simulink model "MATLABxuexiduanluqi"  (R2016a)
settings: Solver=VariableStepAuto  StartTime=0.0  StopTime=0.7  RelTol=1e-3
libraries: powerlib x12
settings Model: Creator=24535  LastModifiedBy=24535

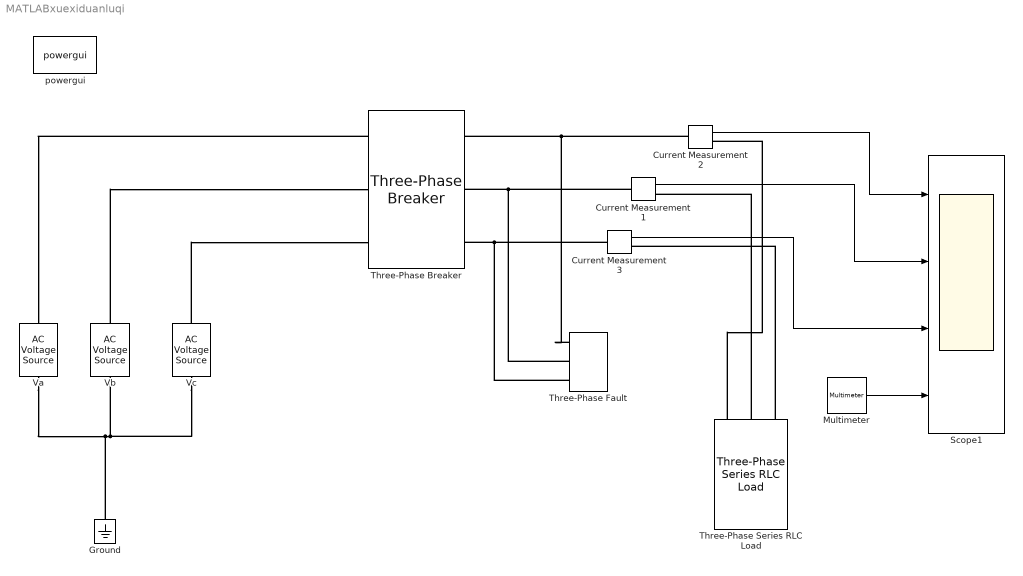
== system MATLABxuexiduanluqi ==
  Current Measurement1 : powerlib/Measurements/Current Measurement  PhasorSimulation=off  OutputType=Complex  PSBequivalent=0
  Current Measurement2 : powerlib/Measurements/Current Measurement  PhasorSimulation=off  OutputType=Complex  PSBequivalent=0
  Current Measurement3 : powerlib/Measurements/Current Measurement  PhasorSimulation=off  OutputType=Complex  PSBequivalent=0
  Ground : powerlib/Elements/Ground  LConnTagsString=a
  Multimeter : powerlib/Measurements/Multimeter  PhasorSimulation=off  OutputType=Complex  sel=7  L=9  Gain=1  yselected={'Ib: Three-Phase Fault/Fault A'};  PSBOutputType=1  PSBequivalent=0  AxesSetting=[0,0.1,-100,100]  Display=0  SavedBlockNames=-11
  Scope1 : Scope  NumInputPorts=4
  Three-Phase Series RLC Load : powerlib/Elements/Three-Phase Series RLC Load  LConnTagsString=A|B|C  Configuration=Y (grounded)  NominalVoltage=5000  Vabc=[1e3 1e3 1e3]  Vabcp=[1e3 1e3 1e3]  NominalFrequency=50  UnbalancedPower=off  ActivePower=1000  InductivePower=330  CapacitivePower=0  Pabc=[10e3 9e3 11e3]  QLabc=[100 90 110]  QCabc=[100 90 110]  Pabcp=[10e3 9e3 11e3]  QLabcp=[100 90 110]  QCabcp=[100 90 110]  Measurements=Branch voltages  LoadType=constant Z
  Three-Phase Breaker : powerlib/Elements/Three-Phase Breaker  InitialState=open  SwitchA=on  SwitchB=on  SwitchC=on  SwitchTimes="[1/50  0.4]"  External=off  BreakerResistance=0.01  SnubberResistance=100  SnubberCapacitance=0.47e-6  Measurements=None
  Three-Phase Fault : powerlib/Elements/Three-Phase Fault  InitialStates=0  FaultA=on  FaultB=on  FaultC=on  GroundFault=on  SwitchTimes="[1/10  3/5]"  External=off  SwitchStatus=NaN  FaultResistance=0.001  GroundResistance=0.01  SnubberResistance=100  SnubberCapacitance=0.47e-6  Measurements=Fault voltages and currents
  Va : powerlib/Electrical Sources/AC Voltage Source  Amplitude=5000  Phase=0  Frequency=50  SampleTime=0  Measurements=None  BusType=swing  Pref=10e3  Qref=0  Qmin=-inf  Qmax=+inf
  Vb : powerlib/Electrical Sources/AC Voltage Source  Amplitude=5000  Phase=120  Frequency=50  SampleTime=0  Measurements=None  BusType=swing  Pref=10e3  Qref=0  Qmin=-inf  Qmax=+inf
  Vc : powerlib/Electrical Sources/AC Voltage Source  Amplitude=5000  Phase=-120  Frequency=50  SampleTime=0  Measurements=None  BusType=swing  Pref=10e3  Qref=0  Qmin=-inf  Qmax=+inf
  powergui : powerlib/powergui  Priority=1  SimulationMode=Continuous  SolverType=Tustin/Backward Euler (TBE)  SampleTime=50e-6  frequency=60  SPID=off  DisableSnubberDevices=off  DisableRonSwitches=off  DisableVfSwitches=off  SwTol=0  DisplayEquations=off  Interpol=off  ExternalGateDelay=off  methode=off  Ts=10  FunctionMessages=off  echomessages=off  HookPort=off  EnableUseOfTLC=off  x0status=blocks  frequencyindice=50  Pbase=100e6  ErrMax=1e-4  Iterations=50  UnitsV=kV  UnitsW=MW  buscounter=0  RestoreLinks=warning  ResistiveCurrentMeasurement=off  Frange=[0:2:500]  Ylog=off  Xlog=on  ShowGrid=off  save=off  variable=ZData  structure=0  ZoomFFT=off  StartTime=0.0  cycles=1  DisplayStyle=1  fundamental=60  FreqAxis=off  MaxFrequency=1000  frequencyindicesteady=1  RmsSteady=1  display=off
  wires:
  Current Measurement2/1 -> Scope1/1
  Current Measurement1/1 -> Scope1/2
  Current Measurement3/1 -> Scope1/3
  Multimeter/1 -> Scope1/4
  connections:
  Current Measurement2/LConn1 -- Three-Phase Fault/LConn1 -- Three-Phase Breaker/RConn1
  Current Measurement1/LConn1 -- Three-Phase Fault/LConn2 -- Three-Phase Breaker/RConn2
  Ground/LConn1 -- Va/LConn1 -- Vc/LConn1 -- Vb/LConn1
  Vc/RConn1 -- Three-Phase Breaker/LConn3
  Vb/RConn1 -- Three-Phase Breaker/LConn2
  Three-Phase Breaker/LConn1 -- Va/RConn1
  Three-Phase Series RLC Load/LConn3 -- Current Measurement3/RConn1
  Three-Phase Series RLC Load/LConn2 -- Current Measurement1/RConn1
  Three-Phase Series RLC Load/LConn1 -- Current Measurement2/RConn1
  Current Measurement3/LConn1 -- Three-Phase Fault/LConn3 -- Three-Phase Breaker/RConn3
